simulink model "refrigeration_PID_room_control_model"  (R2025a)
settings: Solver=VariableStepAuto  StartTime=0.0  StopTime=10.0  RelTol=1e-3
undefined symbols (not defined in the file): Cp, k, Kd, Ki, Kp, m

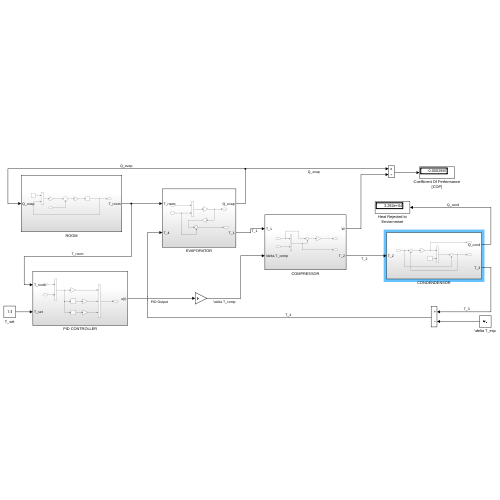
[thumbnail: Simulink's stored preview of the top-level diagram]
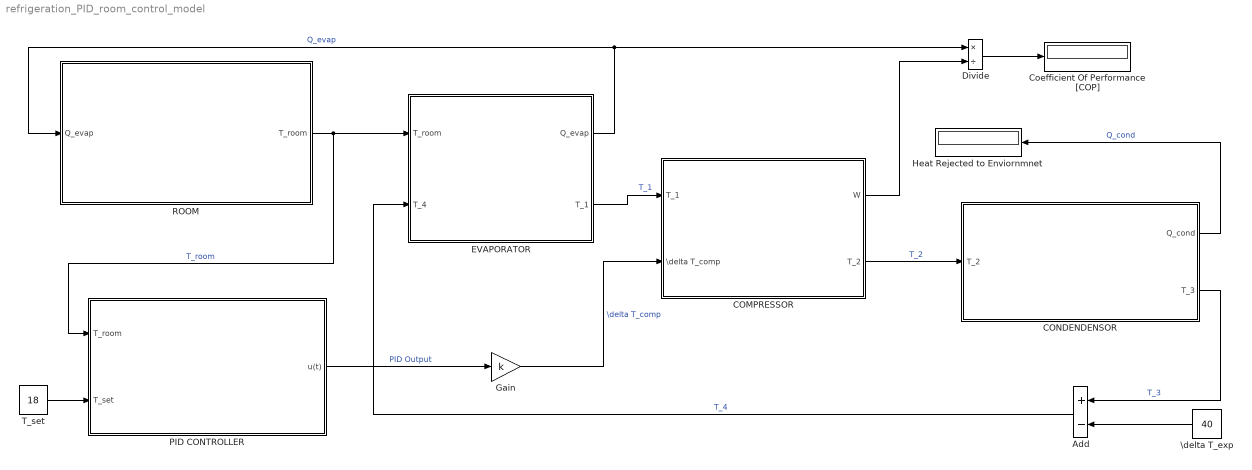
== system refrigeration_PID_room_control_model ==
  Add : Sum  Inputs=+-
  "COMPRESSOR " : Subsystem
  CONDENDENSOR : Subsystem
  Coefficient Of Performance [COP] : Display
  Divide : Product  Inputs=*/
  EVAPORATOR : Subsystem
  Gain : Gain  Gain=k
  Heat Rejected to Enviornmnet : Display
  "PID CONTROLLER " : Subsystem
  "ROOM " : Subsystem
  T_set : Constant  Value=18
  \delta T_exp : Constant  Value=40
  wires:
  EVAPORATOR/2(T_1) -> "COMPRESSOR "/1(T_1)  "T_1"
  "ROOM "/1(T_room) -> "PID CONTROLLER "/1(T_room), EVAPORATOR/1(T_room)  "T_room"
  EVAPORATOR/1(Q_evap) -> "ROOM "/1(Q_evap), Divide/1  "Q_evap"
  "COMPRESSOR "/2(T_2) -> CONDENDENSOR/1(T_2)  "T_2"
  \delta T_exp/1 -> Add/2
  CONDENDENSOR/2(T_3) -> Add/1  "T_3"
  Add/1 -> EVAPORATOR/2(T_4)  "T_4"
  "PID CONTROLLER "/1(u(t)) -> Gain/1  "PID Output"
  Gain/1 -> "COMPRESSOR "/2("\\delta T_comp  ")  "\\delta T_comp"
  T_set/1 -> "PID CONTROLLER "/2(T_set)
  "COMPRESSOR "/1(W) -> Divide/2
  Divide/1 -> Coefficient Of Performance [COP]/1
  CONDENDENSOR/1(Q_cond) -> Heat Rejected to Enviornmnet/1  "Q_cond"

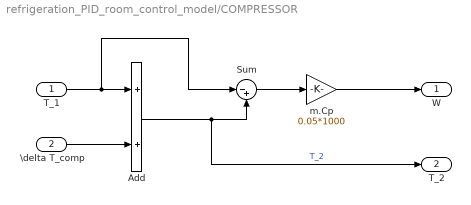
== system refrigeration_PID_room_control_model/COMPRESSOR  ==
  T_1 : Inport
  "\\delta T_comp  " : Inport  Port=2
  Add : Sum
  Sum : Sum  Inputs=|-+
  m.Cp : Gain  Gain=0.05*1000
  W : Outport
  T_2 : Outport  Port=2
  wires:
  T_1/1 -> Sum/1, Add/1
  Sum/1 -> m.Cp/1
  Add/1 -> T_2/1, Sum/2  "T_2"
  m.Cp/1 -> W/1
  "\\delta T_comp  "/1 -> Add/2

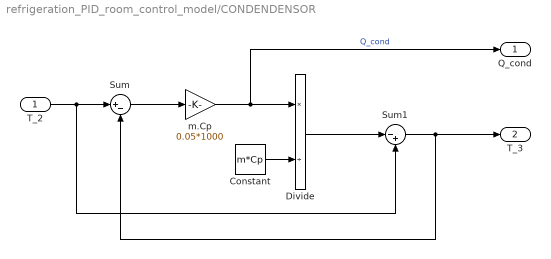
== system refrigeration_PID_room_control_model/CONDENDENSOR ==
  T_2 : Inport
  Constant : Constant  Value=m*Cp
  Divide : Product  Inputs=*/
  Sum : Sum  Inputs=|+-
  Sum1 : Sum  Inputs=|-+
  m.Cp : Gain  Gain=0.05*1000
  Q_cond : Outport
  T_3 : Outport  Port=2
  wires:
  Constant/1 -> Divide/2
  Divide/1 -> Sum1/1
  T_2/1 -> Sum1/2, Sum/1
  m.Cp/1 -> Q_cond/1, Divide/1  "Q_cond"
  Sum/1 -> m.Cp/1
  Sum1/1 -> T_3/1, Sum/2

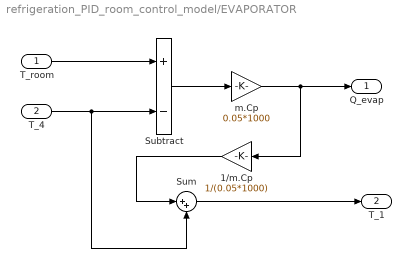
== system refrigeration_PID_room_control_model/EVAPORATOR ==
  T_room : Inport
  T_4 : Inport  Port=2
  1/m.Cp : Gain  Gain=1/(0.05*1000)
  Subtract : Sum  Inputs=+-
  Sum : Sum  Inputs=|++
  m.Cp : Gain  Gain=0.05*1000
  Q_evap : Outport
  T_1 : Outport  Port=2
  wires:
  T_room/1 -> Subtract/1
  1/m.Cp/1 -> Sum/1
  Sum/1 -> T_1/1
  Subtract/1 -> m.Cp/1
  T_4/1 -> Sum/2, Subtract/2
  m.Cp/1 -> Q_evap/1, 1/m.Cp/1

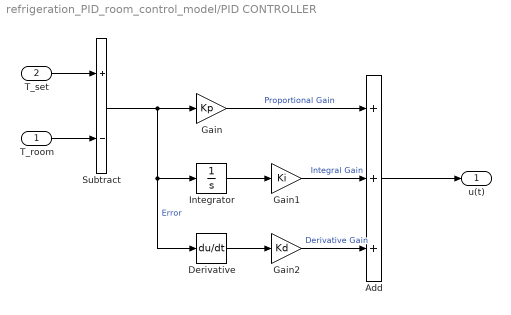
== system refrigeration_PID_room_control_model/PID CONTROLLER  ==
  T_room : Inport
  T_set : Inport  Port=2
  Add : Sum  Inputs=+++
  Derivative : Derivative
  Gain : Gain  Gain=Kp
  Gain1 : Gain  Gain=Ki
  Gain2 : Gain  Gain=Kd
  Integrator : Integrator
  Subtract : Sum  Inputs=+-
  u(t) : Outport
  wires:
  Derivative/1 -> Gain2/1
  T_set/1 -> Subtract/1
  Gain2/1 -> Add/3  "Derivative Gain"
  Gain1/1 -> Add/2  "Integral Gain"
  Subtract/1 -> Gain/1, Integrator/1, Derivative/1  "Error"
  T_room/1 -> Subtract/2
  Integrator/1 -> Gain1/1
  Add/1 -> u(t)/1
  Gain/1 -> Add/1  "Proportional Gain"

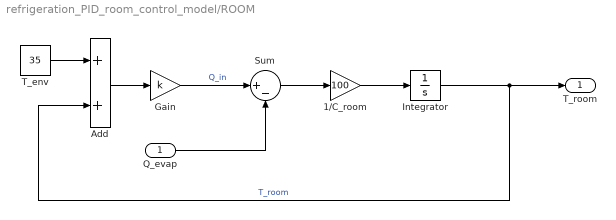
== system refrigeration_PID_room_control_model/ROOM  ==
  Q_evap : Inport
  1/C_room : Gain  Gain=100
  Add : Sum
  Gain : Gain  Gain=k
  Integrator : Integrator
  Sum : Sum  Inputs=|+-
  T_env : Constant  Value=35
  T_room : Outport
  wires:
  Sum/1 -> 1/C_room/1
  Q_evap/1 -> Sum/2
  Add/1 -> Gain/1
  1/C_room/1 -> Integrator/1
  Integrator/1 -> T_room/1, Add/2  "T_room"
  Gain/1 -> Sum/1  "Q_in"
  T_env/1 -> Add/1
